simulink model "testall"  (R2016b)
settings: Solver=VariableStepAuto  StartTime=0.0  StopTime=10.0  FixedStep=1e-7  MinStep=1e-8  RelTol=1e-3
undefined symbols (not defined in the file): fd_d, fd_i, fd_p, Kii, Kpi, me, mj2, mj3, plan, pmsm, q_init, tb, ts, X, Y, Z
libraries: nesl_utility x26, sm_lib x18, fl_lib x11, simulink x8, pe_lib x4, sdl_lib x1, pePwmGeneratorTwoLevel x1
(part 1 of 2)
settings Model: Creator=25097  LastModifiedBy=25097
settings DebuggingCC: AlgebraicLoopMsg=error
settings ExplorerConfigSet: InternalSimMechanicsExplorerSettings="<ExplorerConfiguration><canonicalview>default</canonicalview><AnimationSetting><BasePlaybackSpeed>1.0</BasePlaybackSpeed><PlaybackSpeedFactor>1.0</PlaybackSpeedFactor></AnimationSetting><TilePanel><TileInfo><Tiles Columns=\"1\" Count=\"1\" Rows=\"1\"><Column Left=\"2\" Weight=\"1\"/><Column Left=\"1785\"/><Row Top=\"2\" Weight=\"1\"/><Row Top=\"1285\"/><Tile Height=\"1\" Width=\"1\" X=\"0\" Y=\"0\"/></Tiles></TileInfo><SceneInfo><SceneViewer><BGColor><R>0.60000002384185791</R><G>0.60000002384185791</G><B>0.60000002384185791</B></BGColor><Camera><DoPerspective>off</DoPerspective><Position><X>1.0831826377257374</X><Y>0.51402132352140195</Y><Z>0.67278284493162799</Z></Position><Center><X>0.24747310943545142</X><Y>-0.01628893102971718</Y><Z>0.53009220668623169</Z></Center><Up><X>-0.11789357436721315</X><Y>-0.080526643684547983</Y><Z>0.98975581068252594</Z></Up><ViewLimDist>1</ViewLimDist><YLim>0.67297683779704476</YLim><XLim>0.9370964758649587</XLim></Camera></SceneViewer></SceneInfo></TilePanel><MechEditorPanel><Cameras/><GfxPanelCameraMap/><VideoCreator><PlaybackSpeedRatio>1.0</PlaybackSpeedRatio><FrameRate>30</FrameRate><VideoFormat>MPEG-4</VideoFormat><FrameSize>auto</FrameSize></VideoCreator></MechEditorPanel></ExplorerConfiguration>"

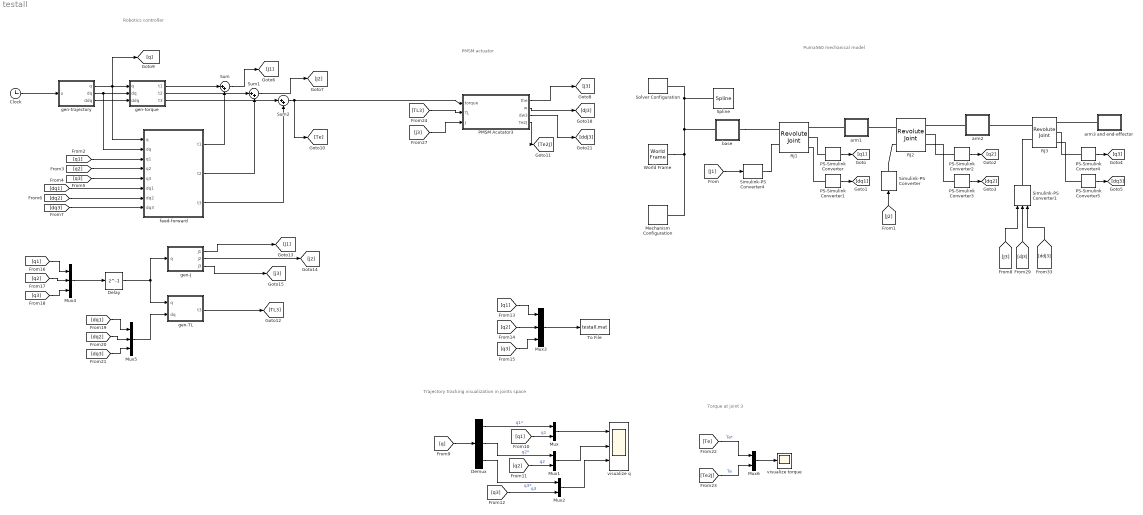
== system testall ==
  note: Robotics controller
  note: Puma560 mechanical model
  note: Trajectory tracking visualization in joints space
  note: PMSM actuator
  note: Torque at joint 3
  Clock : Clock
  Delay : Delay  DelayLength=1
  Demux : Demux  Outputs=3
  Mechanism Configuration : sm_lib/Utilities/Mechanism Configuration  UniformGravity=Constant  GravityVector=[0 0 -9.8]  GravityUnits=m/s^2  LinearizationDelta=0.001
  Mux{,1..2,6} (4 alike) : Mux  Inputs=2
  Mux3 : Mux  Inputs=3
  Mux4 : Mux  Inputs=3
  Mux5 : Mux  Inputs=3
  PMSM Acutator3 : Subsystem
  PS-Simulink Converter : nesl_utility/PS-Simulink Converter  PhysicalDomain=network_engine_domain  SubClassName=ps_output  LeftPortType=input  RightPortType=output  PseudoPeriodic=off  Frequencies=[]  Unit=rad  AffineConversion=off
  PS-Simulink Converter1 : nesl_utility/PS-Simulink Converter  PhysicalDomain=network_engine_domain  SubClassName=ps_output  LeftPortType=input  RightPortType=output  PseudoPeriodic=off  Frequencies=[]  Unit=rad/s  AffineConversion=off
  PS-Simulink Converter2 : nesl_utility/PS-Simulink Converter  PhysicalDomain=network_engine_domain  SubClassName=ps_output  LeftPortType=input  RightPortType=output  PseudoPeriodic=off  Frequencies=[]  Unit=rad  AffineConversion=off
  PS-Simulink Converter3 : nesl_utility/PS-Simulink Converter  PhysicalDomain=network_engine_domain  SubClassName=ps_output  LeftPortType=input  RightPortType=output  PseudoPeriodic=off  Frequencies=[]  Unit=rad/s  AffineConversion=off
  PS-Simulink Converter4 : nesl_utility/PS-Simulink Converter  PhysicalDomain=network_engine_domain  SubClassName=ps_output  LeftPortType=input  RightPortType=output  PseudoPeriodic=off  Frequencies=[]  Unit=rad  AffineConversion=off
  PS-Simulink Converter5 : nesl_utility/PS-Simulink Converter  PhysicalDomain=network_engine_domain  SubClassName=ps_output  LeftPortType=input  RightPortType=output  PseudoPeriodic=off  Frequencies=[]  Unit=rad/s  AffineConversion=off
  RJ1 : sm_lib/Joints/Revolute Joint  SenseConstraintForce=off  SenseConstraintForceX=off  SenseConstraintForceY=off  SenseConstraintForceZ=off  SenseConstraintTorque=off  SenseConstraintTorqueX=off  SenseConstraintTorqueY=off  SenseConstraintTorqueZ=off  SenseTotalForce=off  SenseTotalForceX=off  SenseTotalForceY=off  SenseTotalForceZ=off  SenseTotalTorque=off  SenseTotalTorqueX=off  SenseTotalTorqueY=off  SenseTotalTorqueZ=off  CompositeWrenchDir=FollowerOnBase  CompositeWrenchFrame=BaseFrame  EquilibriumPosition=0  EquilibriumPositionUnits=deg  SpringStiffness=0  SpringStiffnessUnits=N*m/deg  DampingCoefficient=0  DampingCoefficientUnits=N*m/(deg/s)  TorqueActuationMode=InputTorque  MotionActuationMode=ComputedMotion  SensePosition=on  SenseVelocity=on  SenseAcceleration=off  SenseTorqueForce=off  PositionTargetSpecify=off  PositionTargetPriority=High  PositionTargetValue=0  PositionTargetValueUnits=deg  VelocityTargetSpecify=off  VelocityTargetPriority=High  VelocityTargetValue=0  VelocityTargetValueUnits=deg/s
  RJ2 : sm_lib/Joints/Revolute Joint  SenseConstraintForce=off  SenseConstraintForceX=off  SenseConstraintForceY=off  SenseConstraintForceZ=off  SenseConstraintTorque=off  SenseConstraintTorqueX=off  SenseConstraintTorqueY=off  SenseConstraintTorqueZ=off  SenseTotalForce=off  SenseTotalForceX=off  SenseTotalForceY=off  SenseTotalForceZ=off  SenseTotalTorque=off  SenseTotalTorqueX=off  SenseTotalTorqueY=off  SenseTotalTorqueZ=off  CompositeWrenchDir=FollowerOnBase  CompositeWrenchFrame=BaseFrame  EquilibriumPosition=0  EquilibriumPositionUnits=deg  SpringStiffness=0  SpringStiffnessUnits=N*m/deg  DampingCoefficient=0  DampingCoefficientUnits=N*m/(deg/s)  TorqueActuationMode=InputTorque  MotionActuationMode=ComputedMotion  SensePosition=on  SenseVelocity=on  SenseAcceleration=off  SenseTorqueForce=off  PositionTargetSpecify=off  PositionTargetPriority=High  PositionTargetValue=0  PositionTargetValueUnits=deg  VelocityTargetSpecify=off  VelocityTargetPriority=High  VelocityTargetValue=0  VelocityTargetValueUnits=deg/s
  RJ3 : sm_lib/Joints/Revolute Joint  SenseConstraintForce=off  SenseConstraintForceX=off  SenseConstraintForceY=off  SenseConstraintForceZ=off  SenseConstraintTorque=off  SenseConstraintTorqueX=off  SenseConstraintTorqueY=off  SenseConstraintTorqueZ=off  SenseTotalForce=off  SenseTotalForceX=off  SenseTotalForceY=off  SenseTotalForceZ=off  SenseTotalTorque=off  SenseTotalTorqueX=off  SenseTotalTorqueY=off  SenseTotalTorqueZ=off  CompositeWrenchDir=FollowerOnBase  CompositeWrenchFrame=BaseFrame  EquilibriumPosition=0  EquilibriumPositionUnits=deg  SpringStiffness=0  SpringStiffnessUnits=N*m/deg  DampingCoefficient=0  DampingCoefficientUnits=N*m/(deg/s)  TorqueActuationMode=ComputedTorque  MotionActuationMode=InputMotion  SensePosition=on  SenseVelocity=on  SenseAcceleration=off  SenseTorqueForce=off  PositionTargetSpecify=off  PositionTargetPriority=High  PositionTargetValue=0  PositionTargetValueUnits=deg  VelocityTargetSpecify=off  VelocityTargetPriority=High  VelocityTargetValue=0  VelocityTargetValueUnits=deg/s
  Simulink-PS Converter : nesl_utility/Simulink-PS Converter  PhysicalDomain=network_engine_domain  SubClassName=ps_input  LeftPortType=input  RightPortType=output  PseudoPeriodic=off  Frequencies=[]  NoiseDistribution=none  NoiseParameters=[]  Unit=N*m  AffineConversion=off  InputFiltering=off  SimscapeFilterOrder=1  InputFilterTimeConstant=0.001  UdotUserProvided=2
  Simulink-PS Converter1 : nesl_utility/Simulink-PS Converter  PhysicalDomain=network_engine_domain  SubClassName=ps_input  LeftPortType=input  RightPortType=output  PseudoPeriodic=off  Frequencies=[]  NoiseDistribution=none  NoiseParameters=[]  Unit=1  AffineConversion=off  InputFiltering=derivs  SimscapeFilterOrder=1  InputFilterTimeConstant=0.001  UdotUserProvided=2
  Simulink-PS Converter4 : nesl_utility/Simulink-PS Converter  PhysicalDomain=network_engine_domain  SubClassName=ps_input  LeftPortType=input  RightPortType=output  PseudoPeriodic=off  Frequencies=[]  NoiseDistribution=none  NoiseParameters=[]  Unit=N*m  AffineConversion=off  InputFiltering=off  SimscapeFilterOrder=1  InputFilterTimeConstant=0.001  UdotUserProvided=2
  Solver Configuration : nesl_utility/Solver Configuration  PhysicalDomain=network_engine_domain  SubClassName=solver  LeftPortType=input  RightPortType=generic  Accelerate=off  Tones=[]  Harmonics=[]  SimulateNoise=off  Profile=off  UseLocalSampling=off  EnableSwitchedLinearOptims=on  FrequencyDomain=off  UseCCode=off  RelTol=0.001  AbsTol=1e-06  MinStep=1e-09  ToWorkspace=off  RevertToSquareIcSolve=off  NumHomotopyIterations=100  PhasorMode=off  PhasorModeNumHarmonics=1  OverrideAbsTol=off  DoDC=off  ResidualTolerance=1e-09  UseLocalSolver=off  LocalSolverChoice=NE_BACKWARD_EULER_ADVANCER  LocalSolverSampleTime=0.001  DoFixedCost=off  MaxNonlinIter=3  MaxModeIter=2  LinearAlgebra=Sparse  DelaysMemoryBudget=1024  AutomaticFiltering=on  FilteringTimeConstant=0.001
  Spline : sm_lib/Curves and Surfaces/Spline  DataPoints=|  DataPointsUnits=m  EndConditionType=Closed  GraphicType=FromGeometry  MarkerShape=Sphere  MarkerSize=30  GraphicVisPropType=AdvancedVisualProperties  GraphicDiffuseColor=[0.4 1.0 0.2]  GraphicSpecularColor=[0.5 0.5 0.5 1.0]  GraphicAmbientColor=[0.15 0.15 0.15 1.0]  GraphicEmissiveColor=[0.0 0.0 0.0 1.0]  GraphicShininess=100  GraphicOpacity=1.0
      | [0.643990476077583	-0.152700000000000	0.943555134969356
      | 0.643990476077583	-0.215073507245328	0.936999415189498
      | 0.643990476077583	-0.274720992922740	0.917618772262136
      | 0.643990476077583	-0.329035575687742	0.886260233281840
      | 0.643990476077583	-0.375643447643218	0.844294316877014
      | 0.643990476077583	-0.412507621135332	0.793555134969356
      | 0.643990476077583	-0.438016954888546	0.736260233281840
      | 0.643990476077583	-0.451056568610482	0.674913673949652
      | 0.643990476077583	-0.451056568610482	0.612196595989060
      | 0.643990476077583	-0.438016954888546	0.550850036656872
      | 0.643990476077583	-0.412507621135332	0.493555134969356
      | 0.643990476077583	-0.375643447643218	0.442815953061699
      | 0.643990476077583	-0.329035575687742	0.400850036656872
      | 0.643990476077583	-0.274720992922740	0.369491497676576
      | 0.643990476077583	-0.215073507245328	0.350110854749214
      | 0.643990476077583	-0.152700000000000	0.343555134969356
      | 0.643990476077583	-0.0903264927546724	0.350110854749214
      | 0.643990476077583	-0.0306790070772601	0.369491497676576
      | 0.643990476077583	0.0236355756877419	0.400850036656872
      | 0.643990476077583	0.0702434476432181	0.442815953061698
      | 0.643990476077583	0.107107621135332	0.493555134969356
      | 0.643990476077583	0.132616954888546	0.550850036656872
      | 0.643990476077583	0.145656568610482	0.612196595989060
      | 0.643990476077583	0.145656568610482	0.674913673949652
      | 0.643990476077583	0.132616954888546	0.736260233281840
      | 0.643990476077583	0.107107621135332	0.793555134969356
      | 0.643990476077583	0.0702434476432184	0.844294316877013
      | 0.643990476077583	0.0236355756877420	0.886260233281840
      | 0.643990476077583	-0.0306790070772597	0.917618772262136
      | 0.643990476077583	-0.0903264927546720	0.936999415189498]
  Sum : Sum  Inputs=|++
  Sum1 : Sum  Inputs=|++
  Sum2 : Sum  Inputs=|++
  To File : ToFile  Filename=testall.mat  MatrixName=ta  SaveFormat=Timeseries
  World Frame : sm_lib/Frames and Transforms/World Frame
  arm1 : Subsystem
  arm2 : Subsystem
  arm3 and end-effector : Subsystem
  base : Subsystem
  feed-forward : Subsystem
  gen-J : MATLAB Function  TreatAsAtomicUnit=on
  gen-TL : MATLAB Function  TreatAsAtomicUnit=on
  gen-torque : MATLAB Function  TreatAsAtomicUnit=on
  gen-trajectory : MATLAB Function  TreatAsAtomicUnit=on
  visualize torque : Scope
  visualize q : Scope  NumInputPorts=3
  wires:
  Clock/1 -> gen-trajectory/1(u)
  gen-trajectory/1(q) -> [q], feed-forward/1(q), gen-torque/1(q)
  gen-trajectory/2(dq) -> feed-forward/2(dq), gen-torque/2(dq)
  gen-trajectory/3(ddq) -> gen-torque/3(ddq)
  PS-Simulink Converter/1 -> [q1]
  PS-Simulink Converter1/1 -> [dq1]
  PS-Simulink Converter2/1 -> [q2]
  PS-Simulink Converter3/1 -> [dq2]
  PS-Simulink Converter4/1 -> [q3]
  PS-Simulink Converter5/1 -> [dq3]
  [q1] -> feed-forward/3(q1)
  [q2] -> feed-forward/4(q2)
  [q3] -> feed-forward/5(q3)
  [dq1] -> feed-forward/6(dq1)
  [dq2] -> feed-forward/7(dq2)
  [dq3] -> feed-forward/8(dq3)
  gen-torque/1(t1) -> Sum/1
  feed-forward/1(t1) -> Sum/2
  gen-torque/2(t2) -> Sum1/1
  feed-forward/2(t2) -> Sum1/2
  gen-torque/3(t3) -> Sum2/1
  feed-forward/3(t3) -> Sum2/2
  [J1] -> Simulink-PS Converter4/1
  [J2] -> Simulink-PS Converter/1
  [q] -> Demux/1
  Demux/1 -> Mux/1  "q1*"
  [q1] -> Mux/2  "q1"
  Mux/1 -> visualize q/1
  Demux/2 -> Mux1/1  "q2*"
  [q2] -> Mux1/2  "q2"
  Mux1/1 -> visualize q/2
  Mux2/1 -> visualize q/3
  [q3] -> Mux2/2  "q3"
  Demux/3 -> Mux2/1  "q3*"
  [q1] -> Mux3/1
  [q2] -> Mux3/2
  [q3] -> Mux3/3
  Mux3/1 -> To File/1
  [q1] -> Mux4/1
  [q2] -> Mux4/2
  [q3] -> Mux4/3
  [dq1] -> Mux5/1
  [dq2] -> Mux5/2
  [dq3] -> Mux5/3
  Mux5/1 -> gen-TL/2(dq)
  gen-TL/1(t3) -> [TL3]
  PMSM Acutator3/1(the) -> [J3]
  gen-J/1(j1) -> [j1]
  gen-J/2(j2) -> [j2]
  gen-J/3(j3) -> [j3]
  [j3] -> PMSM Acutator3/3("J ")
  PMSM Acutator3/2(w) -> [dJ3]
  PMSM Acutator3/3(dw3) -> [ddJ3]
  Sum/1 -> [J1]
  Sum1/1 -> [J2]
  Sum2/1 -> PMSM Acutator3/1("torque "), [Te]
  [J3] -> Simulink-PS Converter1/1
  [dJ3] -> Simulink-PS Converter1/2
  [ddJ3] -> Simulink-PS Converter1/3
  Mux4/1 -> Delay/1
  [TL3] -> PMSM Acutator3/2(TL)
  Delay/1 -> gen-J/1(q), gen-TL/1(q)
  PMSM Acutator3/4(Te2J) -> [Te2J]
  [Te] -> Mux6/1  "Te*"
  [Te2J] -> Mux6/2  "Te"
  Mux6/1 -> visualize torque/1
  connections:
  Mechanism Configuration/RConn1 -- Spline/LConn1 -- Solver Configuration/RConn1 -- base/LConn1 -- World Frame/RConn1
  arm3 and end-effector/LConn1 -- RJ3/RConn1
  PS-Simulink Converter/LConn1 -- RJ1/RConn2
  arm2/LConn1 -- RJ2/RConn1
  RJ3/LConn1 -- arm2/RConn1
  Simulink-PS Converter4/RConn1 -- RJ1/LConn2
  PS-Simulink Converter3/LConn1 -- RJ2/RConn3
  Simulink-PS Converter1/RConn1 -- RJ3/LConn2
  PS-Simulink Converter5/LConn1 -- RJ3/RConn3
  PS-Simulink Converter4/LConn1 -- RJ3/RConn2
  PS-Simulink Converter1/LConn1 -- RJ1/RConn3
  Simulink-PS Converter/RConn1 -- RJ2/LConn2
  PS-Simulink Converter2/LConn1 -- RJ2/RConn2
  base/RConn1 -- RJ1/LConn1
  arm1/LConn1 -- RJ1/RConn1
  RJ2/LConn1 -- arm1/RConn1

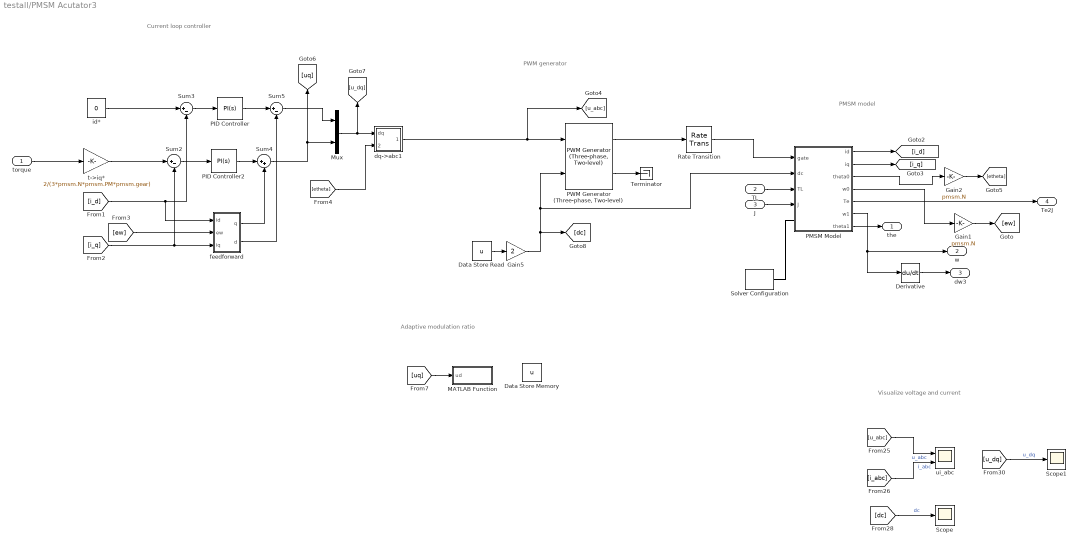
== system testall/PMSM Acutator3 ==
  note: Adaptive modulation ratio
  note: PMSM model
  note: PWM generator
  note: Current loop controller
  note: Visualize voltage and current
  "torque " : Inport
  TL : Inport  Port=2
  "J " : Inport  Port=3
  Data Store Memory : DataStoreMemory  DataStoreName=u  ReadBeforeWriteMsg=warning  WriteAfterWriteMsg=warning  WriteAfterReadMsg=warning  InitialValue=10  ShowAdditionalParam=off  OutDataTypeStr=double
  Data Store Read : DataStoreRead  DataStoreName=u  DataStoreElements=u
  Derivative : Derivative  CoefficientInTFapproximation=1e9
  Gain1 : Gain  Gain=pmsm.N
  Gain2 : Gain  Gain=pmsm.N
  Gain5 : Gain  Gain=2
  MATLAB Function : MATLAB Function  TreatAsAtomicUnit=on
  Mux : Mux  Inputs=2
  PID Controller : simulink/Continuous/PID Controller  Controller=PI  TimeDomain=Continuous-time  SampleTime=-1  IntegratorMethod=Forward Euler  FilterMethod=Forward Euler  Form=Parallel  UseFilter=on  ControllerParametersSource=internal  P=Kpi  I=Kii  D=0  N=100  InitialConditionSource=internal  InitialConditionForIntegrator=0  InitialConditionForFilter=0  ExternalReset=none  LimitOutput=off  UpperSaturationLimit=inf  LowerSaturationLimit=-inf  LinearizeAsGain=on  AntiWindupMode=none  Kb=1  TrackingMode=off  Kt=1  PParamMin=[]  PParamMax=[]  IParamMin=[]  IParamMax=[]  DParamMin=[]  DParamMax=[]  NParamMin=[]  NParamMax=[]  KbParamMin=[]  KbParamMax=[]  KtParamMin=[]  KtParamMax=[]  POutMin=[]  POutMax=[]  IOutMin=[]  IOutMax=[]  DOutMin=[]  DOutMax=[]  NOutMin=[]  NOutMax=[]  KbOutMin=[]  KbOutMax=[]  KtOutMin=[]  KtOutMax=[]  IntegratorOutMin=[]  IntegratorOutMax=[]  FilterOutMin=[]  FilterOutMax=[]  SumOutMin=[]  SumOutMax=[]  SumI1OutMin=[]  SumI1OutMax=[]  SumI2OutMin=[]  SumI2OutMax=[]  SumI3OutMin=[]  SumI3OutMax=[]  SumDOutMin=[]  SumDOutMax=[]  SaturationOutMin=[]  SaturationOutMax=[]  IntegratorContinuousStateAttributes=''  IntegratorStateMustResolveToSignalObject=off  IntegratorRTWStateStorageClass=Auto  FilterContinuousStateAttributes=''  FilterStateMustResolveToSignalObject=off  FilterRTWStateStorageClass=Auto  DifferentiatorICPrevScaledInput=0  DifferentiatorOutMin=[]  DifferentiatorOutMax=[]
  PID Controller2 : simulink/Continuous/PID Controller  Controller=PI  TimeDomain=Continuous-time  SampleTime=-1  IntegratorMethod=Forward Euler  FilterMethod=Forward Euler  Form=Parallel  UseFilter=on  ControllerParametersSource=internal  P=Kpi  I=Kii  D=0  N=100  InitialConditionSource=internal  InitialConditionForIntegrator=0  InitialConditionForFilter=0  ExternalReset=none  LimitOutput=off  UpperSaturationLimit=inf  LowerSaturationLimit=-inf  LinearizeAsGain=on  AntiWindupMode=none  Kb=1  TrackingMode=off  Kt=1  PParamMin=[]  PParamMax=[]  IParamMin=[]  IParamMax=[]  DParamMin=[]  DParamMax=[]  NParamMin=[]  NParamMax=[]  KbParamMin=[]  KbParamMax=[]  KtParamMin=[]  KtParamMax=[]  POutMin=[]  POutMax=[]  IOutMin=[]  IOutMax=[]  DOutMin=[]  DOutMax=[]  NOutMin=[]  NOutMax=[]  KbOutMin=[]  KbOutMax=[]  KtOutMin=[]  KtOutMax=[]  IntegratorOutMin=[]  IntegratorOutMax=[]  FilterOutMin=[]  FilterOutMax=[]  SumOutMin=[]  SumOutMax=[]  SumI1OutMin=[]  SumI1OutMax=[]  SumI2OutMin=[]  SumI2OutMax=[]  SumI3OutMin=[]  SumI3OutMax=[]  SumDOutMin=[]  SumDOutMax=[]  SaturationOutMin=[]  SaturationOutMax=[]  IntegratorContinuousStateAttributes=''  IntegratorStateMustResolveToSignalObject=off  IntegratorRTWStateStorageClass=Auto  FilterContinuousStateAttributes=''  FilterStateMustResolveToSignalObject=off  FilterRTWStateStorageClass=Auto  DifferentiatorICPrevScaledInput=0  DifferentiatorOutMin=[]  DifferentiatorOutMax=[]
  PMSM Model : Subsystem
      settings: MinAlgLoopOccurrences=on
  "PWM Generator (Three-phase, Two-level)" : pePwmGeneratorTwoLevel/PWM Generator (Three-phase, Two-level)  OverrideUsingVariant=NaturalMode  PWMMode=Continuous PWM (CPWM)  CPWMMode=SPWM: sinusoidal PWM  DPWMMode=60 DPWM: 60 degree discontinuous PWM  fsw=fpwm  Ts=ts
      settings: SamplingMode=Natural
  Rate Transition : RateTransition
  Scope : Scope
  Scope1 : Scope
  Solver Configuration : nesl_utility/Solver Configuration  PhysicalDomain=network_engine_domain  SubClassName=solver  LeftPortType=input  RightPortType=generic  Accelerate=off  Tones=[]  Harmonics=[]  SimulateNoise=off  Profile=off  UseLocalSampling=off  EnableSwitchedLinearOptims=on  FrequencyDomain=off  UseCCode=off  RelTol=0.001  AbsTol=1e-06  MinStep=1e-09  ToWorkspace=off  RevertToSquareIcSolve=off  NumHomotopyIterations=100  PhasorMode=off  PhasorModeNumHarmonics=1  OverrideAbsTol=off  DoDC=off  ResidualTolerance=1e-07  UseLocalSolver=off  LocalSolverChoice=NE_BACKWARD_EULER_ADVANCER  LocalSolverSampleTime=1e-6  DoFixedCost=off  MaxNonlinIter=3  MaxModeIter=2  LinearAlgebra=Sparse  DelaysMemoryBudget=1024  AutomaticFiltering=on  FilteringTimeConstant=0.001
  Sum2 : Sum  Inputs=|+-
  Sum3 : Sum  Inputs=|+-
  Sum4 : Sum  Inputs=|++
  Sum5 : Sum  Inputs=|+-
  Terminator : Terminator
  dq->abc1 : Subsystem
  "feedforward " : Subsystem
  id* : Constant  Value=0
  t->iq* : Gain  Gain=2/(3*pmsm.N*pmsm.PM*pmsm.gear)
  ui_abc : Scope  NumInputPorts=2
  the : Outport
  w : Outport  Port=2
  dw3 : Outport  Port=3
  Te2J : Outport  Port=4
  wires:
  PMSM Model/7(theta1) -> the/1
  PMSM Model/6(w1) -> w/1, Derivative/1
  Sum2/1 -> PID Controller2/1
  [ew] -> "feedforward "/2(ew)
  Sum3/1 -> PID Controller/1
  PID Controller/1 -> Sum5/1
  Sum4/1 -> Mux/2, [uq]
  "feedforward "/1(q) -> Sum4/2
  Sum5/1 -> Mux/1
  id*/1 -> Sum3/1
  PID Controller2/1 -> Sum4/1
  "feedforward "/2(d) -> Sum5/2
  dq->abc1/1(abc) -> [u_abc], "PWM Generator (Three-phase, Two-level)"/1
  PMSM Model/5("Te ") -> Te2J/1
  Mux/1 -> dq->abc1/1(dq), [u_dq]
  "PWM Generator (Three-phase, Two-level)"/1 -> Rate Transition/1
  Data Store Read/1 -> Gain5/1
  "PWM Generator (Three-phase, Two-level)"/2 -> Terminator/1
  TL/1 -> PMSM Model/3(TL)
  Gain5/1 -> [dc], "PWM Generator (Three-phase, Two-level)"/2, PMSM Model/2(dc)
  PMSM Model/3(theta0) -> Gain2/1
  PMSM Model/1(id) -> [i_d]
  PMSM Model/4(w0) -> Gain1/1
  Gain1/1 -> [ew]
  [etheta] -> dq->abc1/2("theta ")
  Gain2/1 -> [etheta]
  [uq] -> MATLAB Function/1(ud)
  [i_d] -> "feedforward "/1("id "), Sum3/2
  [i_q] -> "feedforward "/3(iq), Sum2/2
  Rate Transition/1 -> PMSM Model/1("gate ")
  PMSM Model/2(iq) -> [i_q]
  t->iq*/1 -> Sum2/1
  "torque "/1 -> t->iq*/1
  "J "/1 -> PMSM Model/4(J)
  Derivative/1 -> dw3/1
  [u_abc] -> ui_abc/1  "u_abc"
  [i_abc] -> ui_abc/2  "i_abc"
  [dc] -> Scope/1  "dc"
  [u_dq] -> Scope1/1  "u_dq"
  connections:
  Solver Configuration/RConn1 -- PMSM Model/LConn1

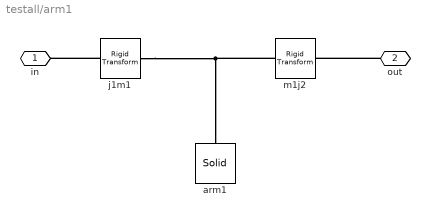
== system testall/arm1 ==
  arm1 : sm_lib/Body Elements/Solid  InertiaType=Custom  Mass=10  MassUnits=kg  CenterOfMass=[0 0 0.102]  CenterOfMassUnits=m  MomentsOfInertia=[0.05 0.05 0.35]  MomentsOfInertiaUnits=kg*m^2  ProductsOfInertia=[0 0 0]  ProductsOfInertiaUnits=kg*m^2  DensityBased=on  Density=8000  DensityUnits=kg/m^3  DoExposeReferenceFrame=on  SerializedFrames=<Frames/>  GraphicType=FromGeometry  MarkerShape=Sphere  MarkerSize=10  GraphicVisPropType=SimpleVisualProperties  GraphicDiffuseColor=[0.2 0.6 1.0]  GraphicSpecularColor=[0.5 0.5 0.5 1.0]  GraphicAmbientColor=[0.15 0.15 0.15 1.0]  GraphicEmissiveColor=[0.0 0.0 0.0 1.0]  GraphicShininess=75  GraphicOpacity=1.0  GeometryShape=FromFile  RectangleSize=[1 1]  RectangleSizeUnits=m  BrickDimensions=[1 1 1]  BrickDimensionUnits=m  CylinderRadius=1  CylinderRadiusUnits=m  CylinderLength=1  CylinderLengthUnits=m  SphereRadius=1  SphereRadiusUnits=m  EllipsoidRadii=[1 1 1]  EllipsoidRadiiUnits=m  ExtrusionCrossSection=[1 1; -1 1; -1 -1; 1 -1]  ExtrusionCrossSectionUnits=m  ExtrusionLength=1  ExtrusionLengthUnits=m  PolygonNumSides=3  PolygonOuterRadius=1  PolygonOuterRadiusUnits=m  ExtGeomFileType=STL  ExtGeomFileName=C:\Users\25097\Desktop\pmsm\puma560_description-master\meshes\puma_link2.stl  ExtGeomFileUnits=in  RevolutionCrossSection=[1 1; 1 -1; 2 -1; 2 1]  RevolutionCrossSectionUnits=m  RevolutionExtent=Full  RevolutionAngle=180  RevolutionAngleUnits=deg
  j1m1 : sm_lib/Frames and Transforms/Rigid Transform  TranslationMethod=Cartesian  TranslationStandardOffset=0  TranslationLengthUnit=m  TranslationStandardAxis=+Z  TranslationCartesianOffset=[0 0.102 0]  TranslationROffset=0  TranslationROffsetUnits=m  TranslationZOffset=0  TranslationZOffsetUnits=m  TranslationThetaOffset=0  TranslationThetaOffsetUnits=deg  RotationMethod=StandardAxis  RotationAngleUnits=deg  RotationStandardAxis=+X  RotationAngle=90  RotationArbitraryAxis=[0 0 1]  FollAlignAxisA=+X  BaseAlignAxisA=+Y  FollAlignAxisB=+Y  BaseAlignAxisB=+Z  RotationSequenceAxes=FollowerAxes  RotationSequence=XYX  RotationSequenceAngles=[0 0 0]  RotationSequenceAnglesUnits=deg  RotationMatrix=[1 0 0; 0 1 0; 0 0 1]
  m1j2 : sm_lib/Frames and Transforms/Rigid Transform  TranslationMethod=StandardAxis  TranslationStandardOffset=0.30  TranslationLengthUnit=m  TranslationStandardAxis=+Z  TranslationCartesianOffset=[0 0.101 0.6718]  TranslationROffset=0  TranslationROffsetUnits=m  TranslationZOffset=0  TranslationZOffsetUnits=m  TranslationThetaOffset=0  TranslationThetaOffsetUnits=deg  RotationMethod=None  RotationAngleUnits=deg  RotationStandardAxis=+X  RotationAngle=90  RotationArbitraryAxis=[0 0 1]  FollAlignAxisA=+X  BaseAlignAxisA=+Y  FollAlignAxisB=+Y  BaseAlignAxisB=+Z  RotationSequenceAxes=FollowerAxes  RotationSequence=XYX  RotationSequenceAngles=[0 0 0]  RotationSequenceAnglesUnits=deg  RotationMatrix=[1 0 0; 0 1 0; 0 0 1]
  in : PMIOPort  Port=1  Side=Left
  out : PMIOPort  Port=2  Side=Right
  connections:
  j1m1/RConn1 -- m1j2/LConn1 -- arm1/RConn1
  j1m1/LConn1 -- in/RConn1
  out/RConn1 -- m1j2/RConn1

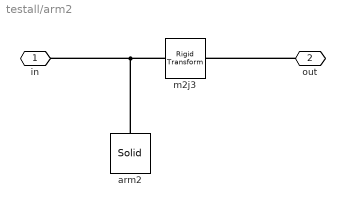
== system testall/arm2 ==
  arm2 : sm_lib/Body Elements/Solid  InertiaType=Custom  Mass=mj2  MassUnits=kg  CenterOfMass=j2c  CenterOfMassUnits=m  MomentsOfInertia=Ij2  MomentsOfInertiaUnits=kg*m^2  ProductsOfInertia=[0 0 0]  ProductsOfInertiaUnits=kg*m^2  DensityBased=on  Density=8000  DensityUnits=kg/m^3  DoExposeReferenceFrame=on  SerializedFrames=<Frames/>  GraphicType=FromGeometry  MarkerShape=Sphere  MarkerSize=10  GraphicVisPropType=SimpleVisualProperties  GraphicDiffuseColor=[0.0 0.8 0.4]  GraphicSpecularColor=[0.5 0.5 0.5 1.0]  GraphicAmbientColor=[0.15 0.15 0.15 1.0]  GraphicEmissiveColor=[0.0 0.0 0.0 1.0]  GraphicShininess=75  GraphicOpacity=1.0  GeometryShape=FromFile  RectangleSize=[1 1]  RectangleSizeUnits=m  BrickDimensions=[1 1 1]  BrickDimensionUnits=m  CylinderRadius=1  CylinderRadiusUnits=m  CylinderLength=1  CylinderLengthUnits=m  SphereRadius=1  SphereRadiusUnits=m  EllipsoidRadii=[1 1 1]  EllipsoidRadiiUnits=m  ExtrusionCrossSection=[1 1; -1 1; -1 -1; 1 -1]  ExtrusionCrossSectionUnits=m  ExtrusionLength=1  ExtrusionLengthUnits=m  PolygonNumSides=3  PolygonOuterRadius=1  PolygonOuterRadiusUnits=m  ExtGeomFileType=STL  ExtGeomFileName=C:\Users\25097\Desktop\pmsm\puma560_description-master\meshes\puma_link3.stl  ExtGeomFileUnits=in  RevolutionCrossSection=[1 1; 1 -1; 2 -1; 2 1]  RevolutionCrossSectionUnits=m  RevolutionExtent=Full  RevolutionAngle=180  RevolutionAngleUnits=deg
  m2j3 : sm_lib/Frames and Transforms/Rigid Transform  TranslationMethod=Cartesian  TranslationStandardOffset=0.30  TranslationLengthUnit=m  TranslationStandardAxis=+Z  TranslationCartesianOffset=[0.4318 -0.0203 -0.0453]  TranslationROffset=0  TranslationROffsetUnits=m  TranslationZOffset=0  TranslationZOffsetUnits=m  TranslationThetaOffset=0  TranslationThetaOffsetUnits=deg  RotationMethod=StandardAxis  RotationAngleUnits=deg  RotationStandardAxis=+Z  RotationAngle=90  RotationArbitraryAxis=[0 0 1]  FollAlignAxisA=+X  BaseAlignAxisA=+Y  FollAlignAxisB=+Y  BaseAlignAxisB=+Z  RotationSequenceAxes=FollowerAxes  RotationSequence=XYX  RotationSequenceAngles=[0 0 0]  RotationSequenceAnglesUnits=deg  RotationMatrix=[1 0 0; 0 1 0; 0 0 1]
  in : PMIOPort  Port=1  Side=Left
  out : PMIOPort  Port=2  Side=Right
  connections:
  out/RConn1 -- m2j3/RConn1
  arm2/RConn1 -- in/RConn1 -- m2j3/LConn1

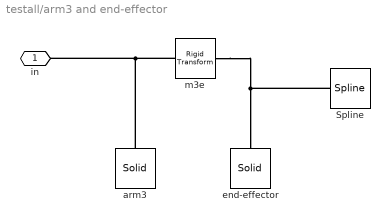
== system testall/arm3 and end-effector ==
  Spline : sm_lib/Curves and Surfaces/Spline  DataPoints=|  DataPointsUnits=m  EndConditionType=Closed  GraphicType=Marker  MarkerShape=Sphere  MarkerSize=30  GraphicVisPropType=SimpleVisualProperties  GraphicDiffuseColor=[1.0 0.2 0.2]  GraphicSpecularColor=[0.5 0.5 0.5 1.0]  GraphicAmbientColor=[0.15 0.15 0.15 1.0]  GraphicEmissiveColor=[0.0 0.0 0.0 1.0]  GraphicShininess=75  GraphicOpacity=1.0
      | [0.643990476077583	-0.152700000000000	0.943555134969356
      | 0.643990476077583	-0.215073507245328	0.936999415189498
      | 0.643990476077583	-0.274720992922740	0.917618772262136
      | 0.643990476077583	-0.329035575687742	0.886260233281840
      | 0.643990476077583	-0.375643447643218	0.844294316877014
      | 0.643990476077583	-0.412507621135332	0.793555134969356
      | 0.643990476077583	-0.438016954888546	0.736260233281840
      | 0.643990476077583	-0.451056568610482	0.674913673949652
      | 0.643990476077583	-0.451056568610482	0.612196595989060
      | 0.643990476077583	-0.438016954888546	0.550850036656872
      | 0.643990476077583	-0.412507621135332	0.493555134969356
      | 0.643990476077583	-0.375643447643218	0.442815953061699
      | 0.643990476077583	-0.329035575687742	0.400850036656872
      | 0.643990476077583	-0.274720992922740	0.369491497676576
      | 0.643990476077583	-0.215073507245328	0.350110854749214
      | 0.643990476077583	-0.152700000000000	0.343555134969356
      | 0.643990476077583	-0.0903264927546724	0.350110854749214
      | 0.643990476077583	-0.0306790070772601	0.369491497676576
      | 0.643990476077583	0.0236355756877419	0.400850036656872
      | 0.643990476077583	0.0702434476432181	0.442815953061698
      | 0.643990476077583	0.107107621135332	0.493555134969356
      | 0.643990476077583	0.132616954888546	0.550850036656872
      | 0.643990476077583	0.145656568610482	0.612196595989060
      | 0.643990476077583	0.145656568610482	0.674913673949652
      | 0.643990476077583	0.132616954888546	0.736260233281840
      | 0.643990476077583	0.107107621135332	0.793555134969356
      | 0.643990476077583	0.0702434476432184	0.844294316877013
      | 0.643990476077583	0.0236355756877420	0.886260233281840
      | 0.643990476077583	-0.0306790070772597	0.917618772262136
      | 0.643990476077583	-0.0903264927546720	0.936999415189498]
  arm3 : sm_lib/Body Elements/Solid  InertiaType=Custom  Mass=mj3  MassUnits=kg  CenterOfMass=[0.05 0 0]  CenterOfMassUnits=m  MomentsOfInertia=Ij3  MomentsOfInertiaUnits=kg*m^2  ProductsOfInertia=[0 0 0]  ProductsOfInertiaUnits=kg*m^2  DensityBased=on  Density=8000  DensityUnits=kg/m^3  DoExposeReferenceFrame=on  SerializedFrames=<Frames/>  GraphicType=FromGeometry  MarkerShape=Sphere  MarkerSize=10  GraphicVisPropType=SimpleVisualProperties  GraphicDiffuseColor=[1.0 0.8 0.6]  GraphicSpecularColor=[0.5 0.5 0.5 1.0]  GraphicAmbientColor=[0.15 0.15 0.15 1.0]  GraphicEmissiveColor=[0.0 0.0 0.0 1.0]  GraphicShininess=75  GraphicOpacity=1.0  GeometryShape=FromFile  RectangleSize=[1 1]  RectangleSizeUnits=m  BrickDimensions=[1 1 1]  BrickDimensionUnits=m  CylinderRadius=1  CylinderRadiusUnits=m  CylinderLength=1  CylinderLengthUnits=m  SphereRadius=1  SphereRadiusUnits=m  EllipsoidRadii=[1 1 1]  EllipsoidRadiiUnits=m  ExtrusionCrossSection=[1 1; -1 1; -1 -1; 1 -1]  ExtrusionCrossSectionUnits=m  ExtrusionLength=1  ExtrusionLengthUnits=m  PolygonNumSides=3  PolygonOuterRadius=1  PolygonOuterRadiusUnits=m  ExtGeomFileType=STL  ExtGeomFileName=C:\Users\25097\Desktop\pmsm\puma560_description-master\meshes\puma_link4.stl  ExtGeomFileUnits=in  RevolutionCrossSection=[1 1; 1 -1; 2 -1; 2 1]  RevolutionCrossSectionUnits=m  RevolutionExtent=Full  RevolutionAngle=180  RevolutionAngleUnits=deg
  end-effector : sm_lib/Body Elements/Solid  InertiaType=PointMass  Mass=me  MassUnits=kg  CenterOfMass=[0 0 0]  CenterOfMassUnits=m  MomentsOfInertia=[1 1 1]  MomentsOfInertiaUnits=kg*m^2  ProductsOfInertia=[1 1 1]  ProductsOfInertiaUnits=kg*m^2  DensityBased=on  Density=8000  DensityUnits=kg/m^3  DoExposeReferenceFrame=on  SerializedFrames=<Frames/>  GraphicType=FromGeometry  MarkerShape=Sphere  MarkerSize=10  GraphicVisPropType=SimpleVisualProperties  GraphicDiffuseColor=[0.5 0.5 0.5]  GraphicSpecularColor=[0.5 0.5 0.5 1.0]  GraphicAmbientColor=[0.15 0.15 0.15 1.0]  GraphicEmissiveColor=[0.0 0.0 0.0 1.0]  GraphicShininess=75  GraphicOpacity=1.0  GeometryShape=FromFile  RectangleSize=[1 1]  RectangleSizeUnits=m  BrickDimensions=[1 1 1]  BrickDimensionUnits=m  CylinderRadius=1  CylinderRadiusUnits=m  CylinderLength=1  CylinderLengthUnits=m  SphereRadius=1  SphereRadiusUnits=m  EllipsoidRadii=[1 1 1]  EllipsoidRadiiUnits=m  ExtrusionCrossSection=[1 1; -1 1; -1 -1; 1 -1]  ExtrusionCrossSectionUnits=m  ExtrusionLength=1  ExtrusionLengthUnits=m  PolygonNumSides=3  PolygonOuterRadius=1  PolygonOuterRadiusUnits=m  ExtGeomFileType=STL  ExtGeomFileName=C:\Users\25097\Desktop\pmsm\puma560_description-master\meshes\puma_link5.stl  ExtGeomFileUnits=in  RevolutionCrossSection=[1 1; 1 -1; 2 -1; 2 1]  RevolutionCrossSectionUnits=m  RevolutionExtent=Full  RevolutionAngle=180  RevolutionAngleUnits=deg
  m3e : sm_lib/Frames and Transforms/Rigid Transform  TranslationMethod=StandardAxis  TranslationStandardOffset=0.361  TranslationLengthUnit=m  TranslationStandardAxis=+X  TranslationCartesianOffset=[0.4318 -0.0203 -0.0453]  TranslationROffset=0  TranslationROffsetUnits=m  TranslationZOffset=0  TranslationZOffsetUnits=m  TranslationThetaOffset=0  TranslationThetaOffsetUnits=deg  RotationMethod=AlignedAxes  RotationAngleUnits=deg  RotationStandardAxis=+Z  RotationAngle=90  RotationArbitraryAxis=[0 0 1]  FollAlignAxisA=+Z  BaseAlignAxisA=+X  FollAlignAxisB=+X  BaseAlignAxisB=-Z  RotationSequenceAxes=FollowerAxes  RotationSequence=XYX  RotationSequenceAngles=[0 0 0]  RotationSequenceAnglesUnits=deg  RotationMatrix=[1 0 0; 0 1 0; 0 0 1]
  "in " : PMIOPort  Port=1  Side=Left
  connections:
  m3e/RConn1 -- end-effector/RConn1 -- Spline/LConn1
  m3e/LConn1 -- "in "/RConn1 -- arm3/RConn1

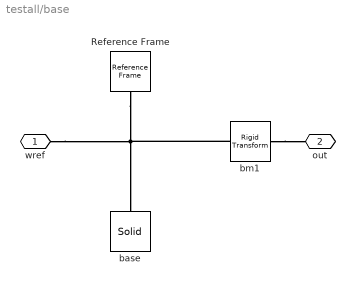
== system testall/base ==
  Reference Frame : sm_lib/Frames and Transforms/Reference Frame
  base : sm_lib/Body Elements/Solid  InertiaType=Custom  Mass=200  MassUnits=kg  CenterOfMass=[0 0 0]  CenterOfMassUnits=m  MomentsOfInertia=[1 1 1]  MomentsOfInertiaUnits=kg*m^2  ProductsOfInertia=[1 1 1]  ProductsOfInertiaUnits=kg*m^2  DensityBased=on  Density=8000  DensityUnits=kg/m^3  DoExposeReferenceFrame=on  SerializedFrames=<Frames/>  GraphicType=FromGeometry  MarkerShape=Sphere  MarkerSize=10  GraphicVisPropType=SimpleVisualProperties  GraphicDiffuseColor=[0.5 0.5 0.5]  GraphicSpecularColor=[0.5 0.5 0.5 1.0]  GraphicAmbientColor=[0.15 0.15 0.15 1.0]  GraphicEmissiveColor=[0.0 0.0 0.0 1.0]  GraphicShininess=75  GraphicOpacity=1.0  GeometryShape=FromFile  RectangleSize=[1 1]  RectangleSizeUnits=m  BrickDimensions=[1 1 1]  BrickDimensionUnits=m  CylinderRadius=1  CylinderRadiusUnits=m  CylinderLength=1  CylinderLengthUnits=m  SphereRadius=1  SphereRadiusUnits=m  EllipsoidRadii=[1 1 1]  EllipsoidRadiiUnits=m  ExtrusionCrossSection=[1 1; -1 1; -1 -1; 1 -1]  ExtrusionCrossSectionUnits=m  ExtrusionLength=1  ExtrusionLengthUnits=m  PolygonNumSides=3  PolygonOuterRadius=1  PolygonOuterRadiusUnits=m  ExtGeomFileType=STL  ExtGeomFileName=C:\Users\25097\Desktop\pmsm\puma560_description-master\meshes\puma_link1.stl  ExtGeomFileUnits=in  RevolutionCrossSection=[1 1; 1 -1; 2 -1; 2 1]  RevolutionCrossSectionUnits=m  RevolutionExtent=Full  RevolutionAngle=180  RevolutionAngleUnits=deg
  bm1 : sm_lib/Frames and Transforms/Rigid Transform  TranslationMethod=Cartesian  TranslationStandardOffset=0.6718  TranslationLengthUnit=m  TranslationStandardAxis=+Z  TranslationCartesianOffset=[0 0 0.6718]  TranslationROffset=0  TranslationROffsetUnits=m  TranslationZOffset=0  TranslationZOffsetUnits=m  TranslationThetaOffset=0  TranslationThetaOffsetUnits=deg  RotationMethod=None  RotationAngleUnits=deg  RotationStandardAxis=+X  RotationAngle=90  RotationArbitraryAxis=[0 0 1]  FollAlignAxisA=+X  BaseAlignAxisA=+Y  FollAlignAxisB=+Y  BaseAlignAxisB=+Z  RotationSequenceAxes=FollowerAxes  RotationSequence=XYX  RotationSequenceAngles=[0 0 0]  RotationSequenceAnglesUnits=deg  RotationMatrix=[1 0 0; 0 1 0; 0 0 1]
  wref : PMIOPort  Port=1  Side=Left
  out : PMIOPort  Port=2  Side=Right
  connections:
  bm1/RConn1 -- out/RConn1
  bm1/LConn1 -- base/RConn1 -- wref/RConn1 -- Reference Frame/RConn1

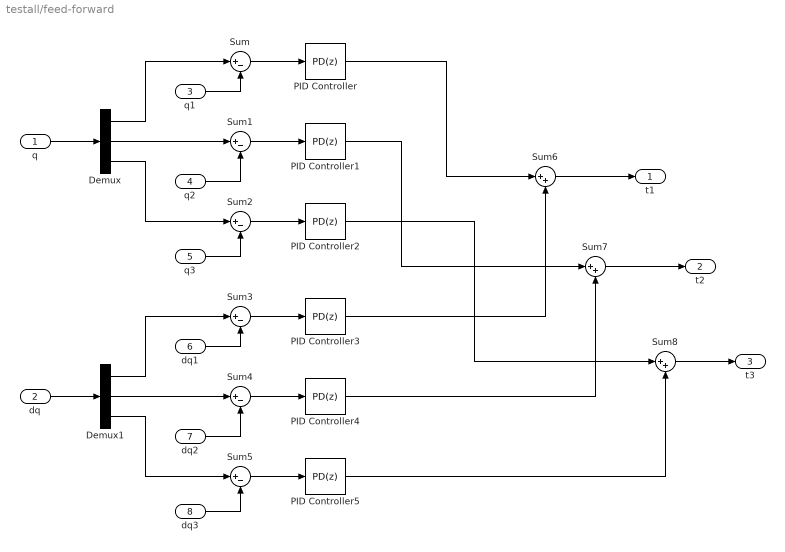
== system testall/feed-forward ==
  q : Inport
  dq : Inport  Port=2
  q1 : Inport  Port=3
  q2 : Inport  Port=4
  q3 : Inport  Port=5
  dq1 : Inport  Port=6
  dq2 : Inport  Port=7
  dq3 : Inport  Port=8
  Demux : Demux  Outputs=3
  Demux1 : Demux  Outputs=3
  PID Controller{,1..5} (6 alike) : simulink/Continuous/PID Controller  Controller=PD  TimeDomain=Discrete-time  SampleTime=-1  IntegratorMethod=Forward Euler  FilterMethod=Forward Euler  Form=Parallel  UseFilter=on  ControllerParametersSource=internal  P=fd_p  I=fd_i  D=fd_d  N=100  InitialConditionSource=internal  InitialConditionForIntegrator=0  InitialConditionForFilter=0  ExternalReset=none  LimitOutput=off  UpperSaturationLimit=inf  LowerSaturationLimit=-inf  LinearizeAsGain=on  AntiWindupMode=none  Kb=1  TrackingMode=off  Kt=1  PParamMin=[]  PParamMax=[]  IParamMin=[]  IParamMax=[]  DParamMin=[]  DParamMax=[]  NParamMin=[]  NParamMax=[]  KbParamMin=[]  KbParamMax=[]  KtParamMin=[]  KtParamMax=[]  POutMin=[]  POutMax=[]  IOutMin=[]  IOutMax=[]  DOutMin=[]  DOutMax=[]  NOutMin=[]  NOutMax=[]  KbOutMin=[]  KbOutMax=[]  KtOutMin=[]  KtOutMax=[]  IntegratorOutMin=[]  IntegratorOutMax=[]  FilterOutMin=[]  FilterOutMax=[]  SumOutMin=[]  SumOutMax=[]  SumI1OutMin=[]  SumI1OutMax=[]  SumI2OutMin=[]  SumI2OutMax=[]  SumI3OutMin=[]  SumI3OutMax=[]  SumDOutMin=[]  SumDOutMax=[]  SaturationOutMin=[]  SaturationOutMax=[]  IntegratorContinuousStateAttributes=''  IntegratorStateMustResolveToSignalObject=off  IntegratorRTWStateStorageClass=Auto  FilterContinuousStateAttributes=''  FilterStateMustResolveToSignalObject=off  FilterRTWStateStorageClass=Auto  DifferentiatorICPrevScaledInput=0  DifferentiatorOutMin=[]  DifferentiatorOutMax=[]
  Sum{,1..5} (6 alike) : Sum  Inputs=|+-
  Sum6 : Sum  Inputs=|++
  Sum7 : Sum  Inputs=|++
  Sum8 : Sum  Inputs=|++
  t1 : Outport
  t2 : Outport  Port=2
  t3 : Outport  Port=3
  wires:
  q/1 -> Demux/1
  dq/1 -> Demux1/1
  Demux/1 -> Sum/1
  Demux/2 -> Sum1/1
  Demux/3 -> Sum2/1
  q1/1 -> Sum/2
  q2/1 -> Sum1/2
  q3/1 -> Sum2/2
  Sum/1 -> PID Controller/1
  Sum1/1 -> PID Controller1/1
  Sum2/1 -> PID Controller2/1
  Demux1/1 -> Sum3/1
  Demux1/2 -> Sum4/1
  Demux1/3 -> Sum5/1
  dq1/1 -> Sum3/2
  dq2/1 -> Sum4/2
  dq3/1 -> Sum5/2
  Sum3/1 -> PID Controller3/1
  Sum4/1 -> PID Controller4/1
  Sum5/1 -> PID Controller5/1
  PID Controller/1 -> Sum6/1
  PID Controller3/1 -> Sum6/2
  PID Controller1/1 -> Sum7/1
  PID Controller4/1 -> Sum7/2
  PID Controller2/1 -> Sum8/1
  PID Controller5/1 -> Sum8/2
  Sum6/1 -> t1/1
  Sum7/1 -> t2/1
  Sum8/1 -> t3/1

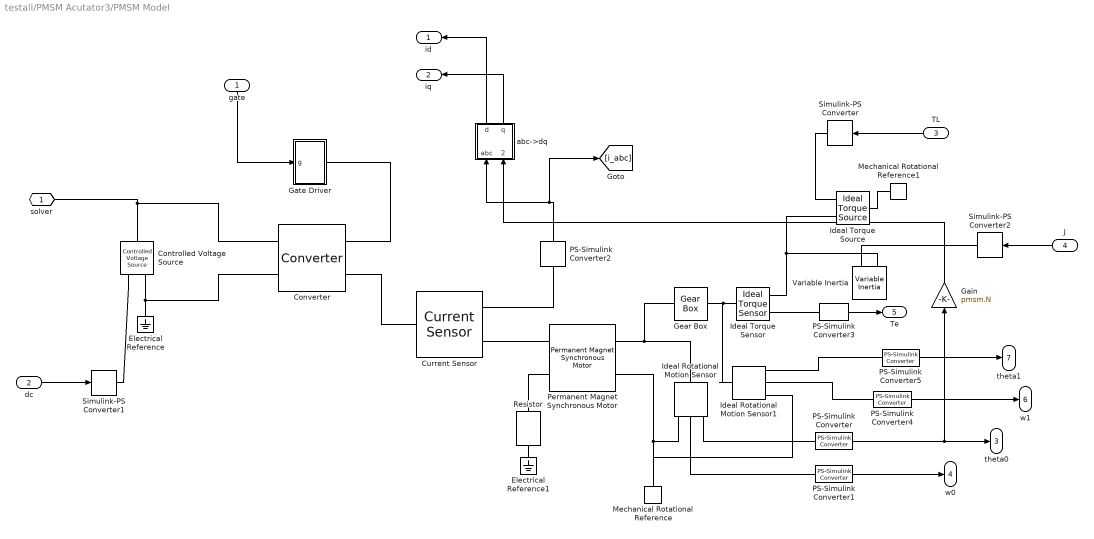
== system testall/PMSM Acutator3/PMSM Model ==
  "gate " : Inport
  dc : Inport  Port=2
  TL : Inport  Port=3
  J : Inport  Port=4
  Controlled Voltage Source : fl_lib/Electrical/Electrical Sources/Controlled Voltage Source
  Converter : pe_lib/Semiconductors/Converter  device_type=2  Vf=0.8 V  Ron=0.001 Ohm  Rds=0.001 Ohm  Goff=1e-8 1/Ohm  Vth=0.5 V  Vgt=1 V  Vgt_off=-1 V  Ih=1 A  diode_param=1  diode_Vf=0.8 V  diode_Ron=0.001 Ohm  diode_Goff=1e-5 1/Ohm  diode_C=50 nF  diode_iRM=-235 A  diode_iF=300 A  diode_idot=-50 A/us  diode_trr_param=1  diode_trr_factor=3  diode_trr=15 us  diode_Qrr=1.5e+3 s*uA  snubber_type=0  Rs=0.1 Ohm  Cs=1e-7 F
  Current Sensor : pe_lib/Sensors/Current Sensor
  Electrical Reference : fl_lib/Electrical/Electrical Elements/Electrical Reference
  Electrical Reference1 : fl_lib/Electrical/Electrical Elements/Electrical Reference
  Gain : Gain  Gain=pmsm.N
  Gate Driver : Subsystem
  Gear Box : fl_lib/Mechanical/Mechanisms/Gear Box  ratio=pmsm.gear  t_in_specify=off  t_in_priority=None  t_in=0 N*m  t_out_specify=off  t_out_priority=None  t_out=0 N*m
  Ideal Rotational Motion Sensor : fl_lib/Mechanical/Mechanical Sensors/Ideal Rotational Motion Sensor  offset=0 rad
  Ideal Rotational Motion Sensor1 : fl_lib/Mechanical/Mechanical Sensors/Ideal Rotational Motion Sensor  offset=0 rad
  Ideal Torque Sensor : fl_lib/Mechanical/Mechanical Sensors/Ideal Torque Sensor
  Ideal Torque Source : fl_lib/Mechanical/Mechanical Sources/Ideal Torque Source
  Mechanical Rotational Reference : fl_lib/Mechanical/Rotational Elements/Mechanical Rotational Reference
  Mechanical Rotational Reference1 : fl_lib/Mechanical/Rotational Elements/Mechanical Rotational Reference
  PS-Simulink Converter{,1..3,5} (5 alike) : nesl_utility/PS-Simulink Converter  PhysicalDomain=network_engine_domain  SubClassName=ps_output  LeftPortType=input  RightPortType=output  PseudoPeriodic=off  Frequencies=[]  Unit=1  AffineConversion=off
  PS-Simulink Converter4 : nesl_utility/PS-Simulink Converter  PhysicalDomain=network_engine_domain  SubClassName=ps_output  LeftPortType=input  RightPortType=output  PseudoPeriodic=off  Frequencies=[]  Unit=rad/s  AffineConversion=off
  Permanent Magnet Synchronous Motor : pe_lib/Machines/Permanent Magnet Rotor/Permanent Magnet Synchronous Motor  nPolePairs=pmsm.N  pm_flux_linkage=pmsm.PM Wb  stator_param=1  Ld=pmsm.Ld H  Lq=pmsm.Ld H  L0=pmsm.Ld H  Ls=0.0002 H  Lm=0.00002 H  Ms=0.00002 H  Rs=pmsm.Rs Ohm  initial_currents=[0.0, 0.0, 0.0] A  axes_param=2  angular_position0=0 rad  rotor_offset=-pi / 2 rad  shift_3ph=[nan, nan, nan] rad  sqrt2OverSqrt3=nan  oneOverSqrt2=nan  twoPiOver3=nan  Lmin=1e-9 H
  Resistor : fl_lib/Electrical/Electrical Elements/Resistor  R=1e9 Ohm  i_specify=off  i_priority=None  i=0 A  v_specify=off  v_priority=None  v=0 V
  Simulink-PS Converter : nesl_utility/Simulink-PS Converter  PhysicalDomain=network_engine_domain  SubClassName=ps_input  LeftPortType=input  RightPortType=output  PseudoPeriodic=off  Frequencies=[]  NoiseDistribution=none  NoiseParameters=[]  Unit=1  AffineConversion=off  InputFiltering=off  SimscapeFilterOrder=1  InputFilterTimeConstant=0.001  UdotUserProvided=1
  Simulink-PS Converter1 : nesl_utility/Simulink-PS Converter  PhysicalDomain=network_engine_domain  SubClassName=ps_input  LeftPortType=input  RightPortType=output  PseudoPeriodic=off  Frequencies=[]  NoiseDistribution=none  NoiseParameters=[]  Unit=V  AffineConversion=off  InputFiltering=off  SimscapeFilterOrder=1  InputFilterTimeConstant=0.001  UdotUserProvided=1
  Simulink-PS Converter2 : nesl_utility/Simulink-PS Converter  PhysicalDomain=network_engine_domain  SubClassName=ps_input  LeftPortType=input  RightPortType=output  PseudoPeriodic=off  Frequencies=[]  NoiseDistribution=none  NoiseParameters=[]  Unit=kg*m^2  AffineConversion=off  InputFiltering=off  SimscapeFilterOrder=1  InputFilterTimeConstant=0.001  UdotUserProvided=1
  Variable Inertia : sdl_lib/Inertias & Loads/Variable Inertia  minimum_inertia=pmsm.J*pmsm.gear^2 kg*m^2  init_momentum=0 m^2*kg/s
  abc->dq : Subsystem
  "solver " : PMIOPort  Port=1  Side=Left
  id : Outport
  iq : Outport  Port=2
  theta0 : Outport  Port=3
  w0 : Outport  Port=4
  "Te " : Outport  Port=5
  w1 : Outport  Port=6
  theta1 : Outport  Port=7
  wires:
  PS-Simulink Converter/1 -> Gain/1, theta0/1
  PS-Simulink Converter2/1 -> [i_abc], abc->dq/1(abc)
  PS-Simulink Converter1/1 -> w0/1
  abc->dq/1(d) -> id/1
  abc->dq/2(q) -> iq/1
  PS-Simulink Converter3/1 -> "Te "/1
  Gain/1 -> abc->dq/2(theta)
  "gate "/1 -> Gate Driver/1(g)
  dc/1 -> Simulink-PS Converter1/1
  TL/1 -> Simulink-PS Converter/1
  PS-Simulink Converter4/1 -> w1/1
  PS-Simulink Converter5/1 -> theta1/1
  J/1 -> Simulink-PS Converter2/1
  connections:
  Electrical Reference/LConn1 -- Controlled Voltage Source/RConn2 -- Converter/RConn2
  Converter/RConn1 -- "solver "/RConn1 -- Controlled Voltage Source/LConn1
  Current Sensor/RConn1 -- PS-Simulink Converter2/LConn1
  Converter/LConn2 -- Current Sensor/LConn1
  Resistor/LConn1 -- Permanent Magnet Synchronous Motor/LConn2
  Current Sensor/RConn2 -- Permanent Magnet Synchronous Motor/LConn1
  Electrical Reference1/LConn1 -- Resistor/RConn1
  Gate Driver/RConn1 -- Converter/LConn1
  Permanent Magnet Synchronous Motor/RConn2 -- Ideal Rotational Motion Sensor/RConn1 -- Ideal Rotational Motion Sensor1/RConn1 -- Mechanical Rotational Reference/LConn1
  Ideal Torque Source/RConn2 -- Ideal Torque Sensor/RConn1 -- Variable Inertia/LConn2
  Ideal Rotational Motion Sensor/RConn3 -- PS-Simulink Converter/LConn1
  Ideal Rotational Motion Sensor/RConn2 -- PS-Simulink Converter1/LConn1
  PS-Simulink Converter3/LConn1 -- Ideal Torque Sensor/RConn2
  Controlled Voltage Source/RConn1 -- Simulink-PS Converter1/RConn1
  Mechanical Rotational Reference1/LConn1 -- Ideal Torque Source/LConn1
  Ideal Torque Source/RConn1 -- Simulink-PS Converter/RConn1
  Permanent Magnet Synchronous Motor/RConn1 -- Ideal Rotational Motion Sensor/LConn1 -- Gear Box/LConn1
  PS-Simulink Converter4/LConn1 -- Ideal Rotational Motion Sensor1/RConn2
  PS-Simulink Converter5/LConn1 -- Ideal Rotational Motion Sensor1/RConn3
  Ideal Torque Sensor/LConn1 -- Gear Box/RConn1 -- Ideal Rotational Motion Sensor1/LConn1
  Simulink-PS Converter2/RConn1 -- Variable Inertia/LConn1

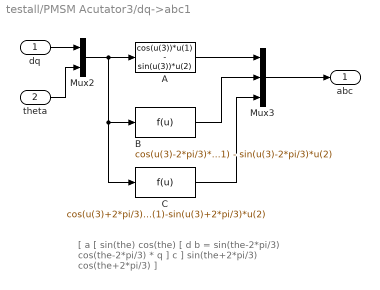
== system testall/PMSM Acutator3/dq->abc1 ==
  note: [ a        [  sin(the)               cos(the)                 [ d
      |
      |   b    =     sin(the-2*pi/3)    cos(the-2*pi/3)    *    q ]
      |
      |   c ]         sin(the+2*pi/3)   cos(the+2*pi/3) ]
  dq : Inport
  "theta " : Inport  Port=2
  A : Fcn  Expr=cos(u(3))*u(1) - sin(u(3))*u(2)
  B : Fcn  Expr=cos(u(3)-2*pi/3)*u(1) - sin(u(3)-2*pi/3)*u(2)
  C : Fcn  Expr=cos(u(3)+2*pi/3)*u(1)-sin(u(3)+2*pi/3)*u(2)
  Mux2 : Mux  Inputs=2
  Mux3 : Mux  Inputs=3
  abc : Outport
  wires:
  Mux3/1 -> abc/1
  C/1 -> Mux3/3
  A/1 -> Mux3/1
  dq/1 -> Mux2/1
  "theta "/1 -> Mux2/2
  Mux2/1 -> C/1, B/1, A/1
  B/1 -> Mux3/2

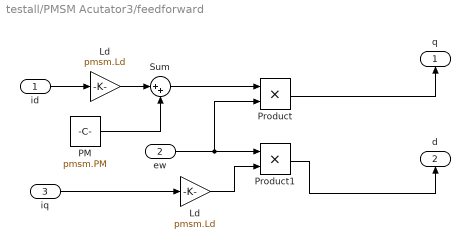
== system testall/PMSM Acutator3/feedforward  ==
  "id " : Inport
  ew : Inport  Port=2
  iq : Inport  Port=3
  Ld : Gain  Gain=pmsm.Ld
  "Ld " : Gain  Gain=pmsm.Ld
  PM : Constant  Value=pmsm.PM
  Product : Product
  Product1 : Product
  Sum : Sum  Inputs=|++
  q : Outport
  d : Outport  Port=2
  wires:
  "id "/1 -> Ld/1
  PM/1 -> Sum/2
  Ld/1 -> Sum/1
  "Ld "/1 -> Product1/2
  Product/1 -> q/1
  Sum/1 -> Product/1
  Product1/1 -> d/1
  iq/1 -> "Ld "/1
  ew/1 -> Product1/1, Product/2

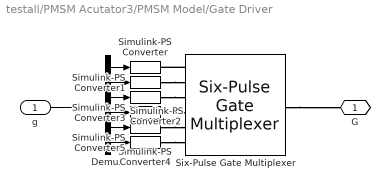
== system testall/PMSM Acutator3/PMSM Model/Gate Driver ==
  g : Inport
  Demux : Demux  Outputs=6
  Simulink-PS Converter{,1..5} (6 alike) : nesl_utility/Simulink-PS Converter  PhysicalDomain=network_engine_domain  SubClassName=ps_input  LeftPortType=input  RightPortType=output  PseudoPeriodic=off  Frequencies=[]  NoiseDistribution=none  NoiseParameters=[]  Unit=1  AffineConversion=off  InputFiltering=off  SimscapeFilterOrder=1  InputFilterTimeConstant=0.001  UdotUserProvided=1
  Six-Pulse Gate Multiplexer : pe_lib/Semiconductors/Six-Pulse Gate Multiplexer  R=0 Ohm
  G : PMIOPort  Port=1  Side=Right
  wires:
  g/1 -> Demux/1
  Demux/1 -> Simulink-PS Converter/1
  Demux/2 -> Simulink-PS Converter1/1
  Demux/3 -> Simulink-PS Converter2/1
  Demux/4 -> Simulink-PS Converter3/1
  Demux/5 -> Simulink-PS Converter4/1
  Demux/6 -> Simulink-PS Converter5/1
  connections:
  Six-Pulse Gate Multiplexer/LConn1 -- Simulink-PS Converter/RConn1
  Simulink-PS Converter1/RConn1 -- Six-Pulse Gate Multiplexer/LConn2
  Simulink-PS Converter2/RConn1 -- Six-Pulse Gate Multiplexer/LConn3
  Simulink-PS Converter3/RConn1 -- Six-Pulse Gate Multiplexer/LConn4
  Simulink-PS Converter4/RConn1 -- Six-Pulse Gate Multiplexer/LConn5
  Simulink-PS Converter5/RConn1 -- Six-Pulse Gate Multiplexer/LConn6
  Six-Pulse Gate Multiplexer/RConn1 -- G/RConn1

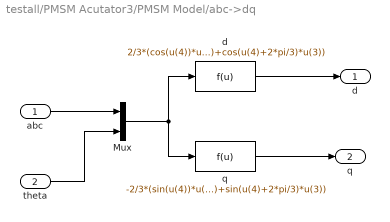
== system testall/PMSM Acutator3/PMSM Model/abc->dq ==
  abc : Inport
  theta : Inport  Port=2
  Mux : Mux  Inputs=2
  "d " : Fcn  Expr=2/3*(cos(u(4))*u(1)+cos(u(4)-2*pi/3)*u(2)+cos(u(4)+2*pi/3)*u(3))
  "q " : Fcn  Expr=-2/3*(sin(u(4))*u(1)+sin(u(4)-2*pi/3)*u(2)+sin(u(4)+2*pi/3)*u(3))
  d : Outport
  q : Outport  Port=2
  wires:
  "d "/1 -> d/1
  "q "/1 -> q/1
  abc/1 -> Mux/1
  Mux/1 -> "q "/1, "d "/1
  theta/1 -> Mux/2
